simulink model "testenv"  (R2022b)
settings: Solver=VariableStepAuto  StartTime=0.0  StopTime=10.0  RelTol=1e-3
values from neighbouring files (symbols this model uses):
  sampleTime = 0.1    [RRT.m]
libraries: mobileRoboticsLib x9
settings Model: Creator=OEM  LastModifiedBy=OEM

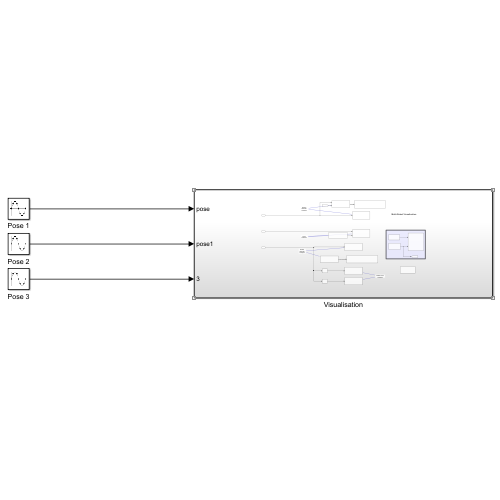
[thumbnail: Simulink's stored preview of the top-level diagram]
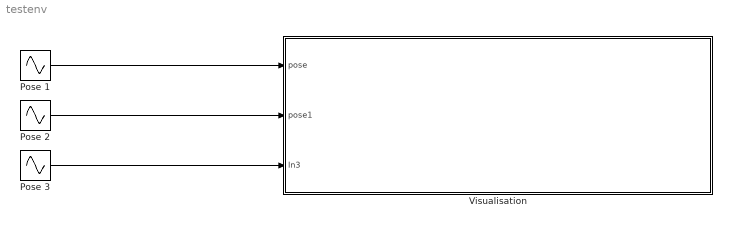
== system testenv ==
  Pose 1 : Sin  SineType=Sample based  Amplitude=[1;1.5;pi/4]  Bias=[2;2;0]  Phase=[0;pi/2;0]  Samples=200  SampleTime=sampleTime
  Pose 2 : Sin  SineType=Sample based  Amplitude=[-1.5;1;2*pi/3]  Bias=[10;10;-pi/3]  Phase=[0;pi/2;0]  Samples=150  SampleTime=sampleTime
  Pose 3 : Sin  SineType=Sample based  Amplitude=[-2;0.5;pi/2]  Bias=[7.75;3;0]  Phase=[-pi/4;0;pi/3]  Samples=160  SampleTime=sampleTime  Offset=[0;50;25]
  Visualisation : Subsystem
  wires:
  Pose 1/1 -> Visualisation/1(pose)
  Pose 2/1 -> Visualisation/2(pose1)
  Pose 3/1 -> Visualisation/3(In3)

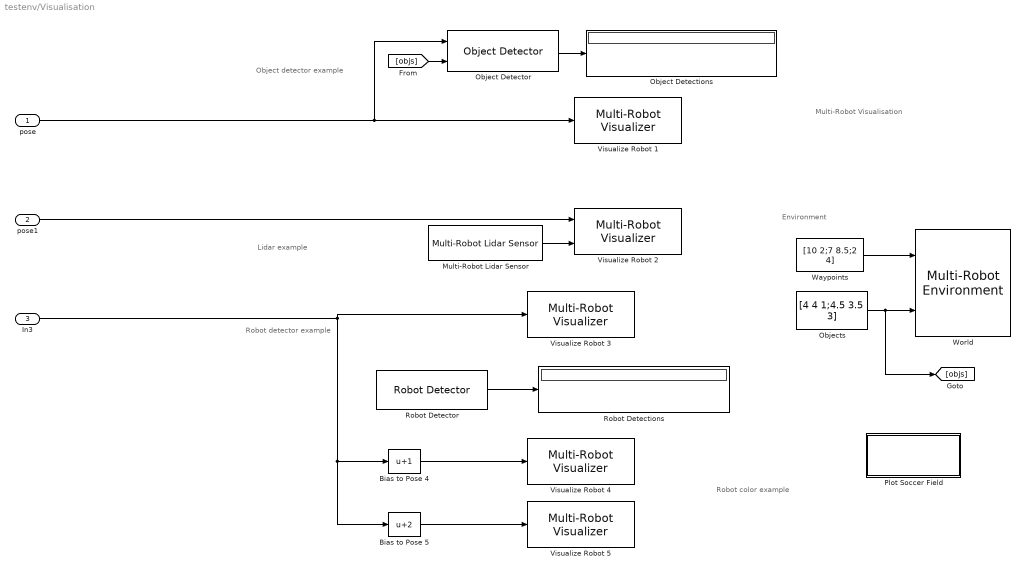
== system testenv/Visualisation ==
  note: Lidar example
  note: Object detector example
  note: Environment
  note: Multi-Robot Visualisation
  note: Robot color example
  note: Robot detector example
  pose : Inport
  pose1 : Inport  Port=2
  In3 : Inport  Port=3
  Bias to Pose 4 : Bias  Bias=1  SaturateOnIntegerOverflow=off
  Bias to Pose 5 : Bias  Bias=2  SaturateOnIntegerOverflow=off
  Multi-Robot Lidar Sensor : mobileRoboticsLib/Environments/Multi-Robot Lidar Sensor  robotIdx=2  mapName=map  sensorOffset=sensorOffset  scanAngles=scanAngles  maxRange=maxRange
      settings: SourceProductName=Mobile Robotics Simulation Toolbox
  Object Detections : Display
  Object Detector : mobileRoboticsLib/Environments/Object Detector  mapName=map  sensorOffset=objDetectorOffset  sensorAngle=objDetectorAngle  fieldOfView=objDetectorFOV  maxRange=objDetectorRange  maxDetections=objDetectorMaxHits  sampleTime=-1
      settings: SourceProductName=Mobile Robotics Simulation Toolbox
  Objects : Constant  Value=[4 4 1;4.5 3.5 3]
  Plot Soccer Field : MATLAB Function  TreatAsAtomicUnit=on
  Robot Detections : Display
  Robot Detector : mobileRoboticsLib/Environments/Robot Detector  mapName=map  robotIdx=3  sensorOffset=[ 0, 0 ]  sensorAngle=0  sensorFOV=pi/3  maxRange=10  maxDetections=3  sampleTime=-1
      settings: SourceProductName=Mobile Robotics Simulation Toolbox
  Visualize Robot 1 : mobileRoboticsLib/Environments/Multi-Robot Visualizer  idx=1  radius=0  robotColor=[0 0 1]  showTraj=on  hasLidar=off  sensorOffset=sensorOffset  scanAngles=scanAngles  maxNumScans=0  hasObjDetector=on  objDetectorOffset=objDetectorOffset  objDetectorAngle=objDetectorAngle  objDetectorFOV=objDetectorFOV  objDetectorMaxRange=objDetectorRange  hasRobotDetector=off  robotDetectorOffset=[0,0]  robotDetectorAngle=0  robotDetectorFOV=pi/3  robotDetectorMaxRange=5  robotDetectorNumDetections=0
      settings: SourceProductName=Mobile Robotics Simulation Toolbox
  Visualize Robot 2 : mobileRoboticsLib/Environments/Multi-Robot Visualizer  idx=2  radius=0.5  robotColor=[0 0 1]  showTraj=on  hasLidar=on  sensorOffset=sensorOffset  scanAngles=scanAngles  maxNumScans=0  hasObjDetector=off  objDetectorOffset=objDetectorOffset  objDetectorAngle=objDetectorAngle  objDetectorFOV=objDetectorFOV  objDetectorMaxRange=objDetectorRange  hasRobotDetector=off  robotDetectorOffset=[0,0]  robotDetectorAngle=0  robotDetectorFOV=pi/3  robotDetectorMaxRange=5  robotDetectorNumDetections=0
      settings: SourceProductName=Mobile Robotics Simulation Toolbox
  Visualize Robot 3 : mobileRoboticsLib/Environments/Multi-Robot Visualizer  idx=3  radius=0.25  robotColor=[0 0 1]  showTraj=on  hasLidar=off  sensorOffset=sensorOffset  scanAngles=scanAngles  maxNumScans=0  hasObjDetector=off  objDetectorOffset=objDetectorOffset  objDetectorAngle=objDetectorAngle  objDetectorFOV=objDetectorFOV  objDetectorMaxRange=objDetectorRange  hasRobotDetector=on  robotDetectorOffset=[0,0]  robotDetectorAngle=0  robotDetectorFOV=pi/3  robotDetectorMaxRange=10  robotDetectorNumDetections=0
      settings: SourceProductName=Mobile Robotics Simulation Toolbox
  Visualize Robot 4 : mobileRoboticsLib/Environments/Multi-Robot Visualizer  idx=4  radius=0.5  robotColor=[0 0.8 0]  showTraj=off  hasLidar=off  sensorOffset=sensorOffset  scanAngles=scanAngles  maxNumScans=0  hasObjDetector=off  objDetectorOffset=objDetectorOffset  objDetectorAngle=objDetectorAngle  objDetectorFOV=objDetectorFOV  objDetectorMaxRange=objDetectorRange  hasRobotDetector=off  robotDetectorOffset=[0,0]  robotDetectorAngle=0  robotDetectorFOV=pi/3  robotDetectorMaxRange=5  robotDetectorNumDetections=0
      settings: SourceProductName=Mobile Robotics Simulation Toolbox
  Visualize Robot 5 : mobileRoboticsLib/Environments/Multi-Robot Visualizer  idx=5  radius=0.25  robotColor=[0.6 0 0]  showTraj=off  hasLidar=off  sensorOffset=sensorOffset  scanAngles=scanAngles  maxNumScans=0  hasObjDetector=off  objDetectorOffset=objDetectorOffset  objDetectorAngle=objDetectorAngle  objDetectorFOV=objDetectorFOV  objDetectorMaxRange=objDetectorRange  hasRobotDetector=off  robotDetectorOffset=[0,0]  robotDetectorAngle=0  robotDetectorFOV=pi/3  robotDetectorMaxRange=5  robotDetectorNumDetections=0
      settings: SourceProductName=Mobile Robotics Simulation Toolbox
  Waypoints : Constant  Value=[10 2;7 8.5;2 4]
  World : mobileRoboticsLib/Environments/Multi-Robot Environment  numRobots=num_robots  mapName=map  showWaypoints=on  showObjects=on  objectColors=[1 0 0;0 1 0;0 0 1]  objectMarkers='so^'  showRobotIds=on  plotSensorLines=on
      settings: SourceProductName=Mobile Robotics Simulation Toolbox
  wires:
  pose/1 -> Object Detector/1, Visualize Robot 1/1
  Waypoints/1 -> World/1
  [objs] -> Object Detector/2
  Robot Detector/1 -> Robot Detections/1
  Objects/1 -> [objs], World/2
  Bias to Pose 4/1 -> Visualize Robot 4/1
  Object Detector/1 -> Object Detections/1
  Bias to Pose 5/1 -> Visualize Robot 5/1
  In3/1 -> Bias to Pose 5/1, Bias to Pose 4/1, Visualize Robot 3/1
  Multi-Robot Lidar Sensor/1 -> Visualize Robot 2/2
  pose1/1 -> Visualize Robot 2/1

== matlab function testenv/Visualisation/Plot Soccer Field ==
function plotSoccerField
% Plots the soccer field once the figure window for the environment has
% been initialized

rectangle('Position',[0 0 11 8])
rectangle('Position',[1 1 9 6])
